simulink model "svm_limiter_test"  (R2015a)
settings: Solver=ode45  StartTime=0.0  StopTime=0.1  RelTol=1e-3
libraries: simulink x1
settings Model: Creator=user  LastModifiedBy=user

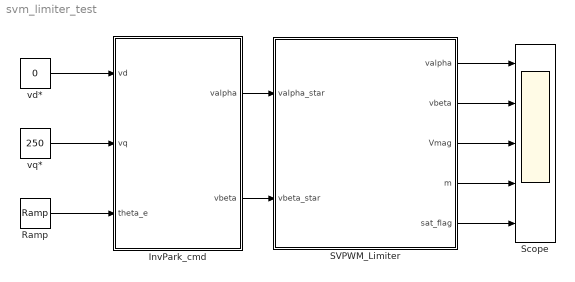
== system svm_limiter_test ==
  InvPark_cmd : MATLAB Function  TreatAsAtomicUnit=on
  Ramp : simulink/Sources/Ramp  slope=20*pi  start=0  X0=0
  SVPWM_Limiter : MATLAB Function  TreatAsAtomicUnit=on
  Scope : Scope  NumInputPorts=5
      settings: YMin=-5~-5~-5~-5~-5  YMax=5~5~5~5~5
  vd* : Constant  Value=0
  vq* : Constant  Value=250
  wires:
  vd*/1 -> InvPark_cmd/1(vd)
  vq*/1 -> InvPark_cmd/2(vq)
  Ramp/1 -> InvPark_cmd/3(theta_e)
  InvPark_cmd/2(vbeta) -> SVPWM_Limiter/2(vbeta_star)
  InvPark_cmd/1(valpha) -> SVPWM_Limiter/1(valpha_star)
  SVPWM_Limiter/1(valpha) -> Scope/1
  SVPWM_Limiter/4(m) -> Scope/4
  SVPWM_Limiter/5(sat_flag) -> Scope/5
  SVPWM_Limiter/3(Vmag) -> Scope/3
  SVPWM_Limiter/2(vbeta) -> Scope/2

== matlab function svm_limiter_test/InvPark_cmd ==
  data: vd input; valpha output; vq input; theta_e input; vbeta output
function [valpha, vbeta] = InvPark_cmd(vd, vq, theta_e)

valpha = vd*cos(theta_e) - vq*sin(theta_e);

vbeta = vd*sin(theta_e) + vq*cos(theta_e);

== matlab function svm_limiter_test/SVPWM_Limiter ==
  data: valpha_star input; valpha output; vbeta_star input; vbeta output; Vmag output; m output; sat_flag output
function [valpha, vbeta, Vmag, m, sat_flag] = SVPWM_Limiter(valpha_star, vbeta_star)

Vmax = 360/sqrt(3);

Vmag = sqrt(valpha_star^2 + vbeta_star^2);

m = Vmag/Vmax;

if Vmag <= Vmax
    valpha = valpha_star;
    vbeta = vbeta_star;
    sat_flag = 0;
else
    scale = Vmax/Vmag;
    valpha = valpha_star*scale;
    vbeta = vbeta_star*scale;
    sat_flag = 1;
end
